simulink model "CubaModelTwoPoint"  (R2016a)
settings: Solver=FixedStepAuto  SolverMode=SingleTasking  StartTime=0.0  StopTime=5  FixedStep=0.001  RelTol=1e-3
values from neighbouring files (symbols this model uses):
  C_K = 2.1e-3    (= 0.0021)    [Init_TwoPoint.m]
  C_R = 2.1268e-5    (= 2.1268e-05)    [Init_TwoPoint.m]
  g = 9.81    [Init_TwoPoint.m]
  l_AB = 0.08455    [Init_TwoPoint.m]
  l_SA = 0.0751442    [Init_TwoPoint.m]
  m_K = 0.294    [Init_TwoPoint.m]
  m_R = 0.1298    [Init_TwoPoint.m]
  O_G_A = O_K_A + m_R * l_AB^2    (= 0.0042279015845)    [Init_TwoPoint.m]
  O_R_B = 0.088e-3    (= 8.8e-05)    [Init_TwoPoint.m]
  phi_K0 = degtorad(1)    [Init_TwoPoint.m]
  phi_K__d0 = degtorad(0)    [Init_TwoPoint.m]
  phi_R0 = degtorad(0)    [Init_TwoPoint.m]
  phi_R__d0 = degtorad(0)    [Init_TwoPoint.m]
  T_M_m = 12.4e-3    (= 0.0124)    [Init_TwoPoint.m]
undefined symbols (not defined in the file or in its folder): degtorad
libraries: simulink x1
settings Model: Creator=michael  LastModifiedBy=ich

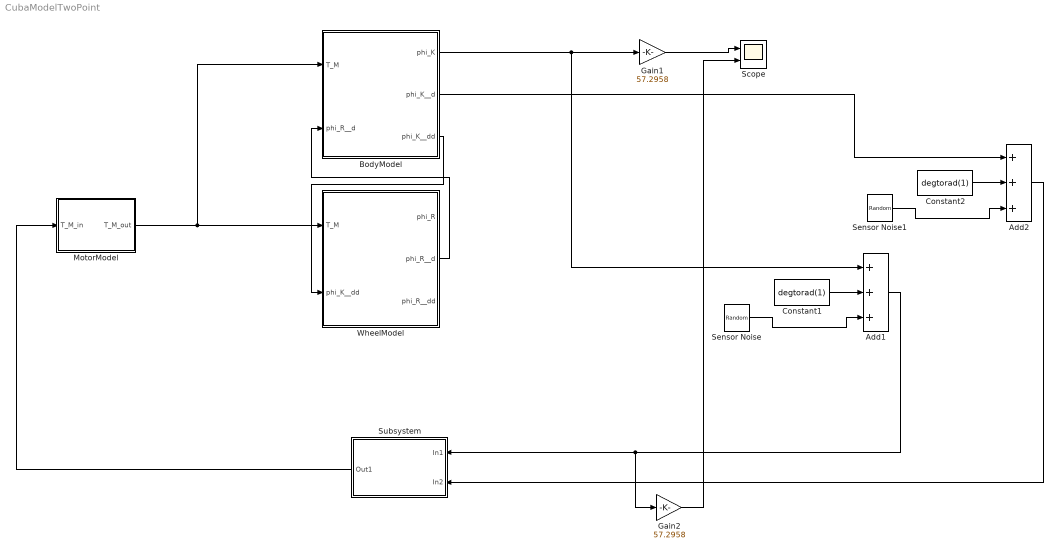
== system CubaModelTwoPoint ==
  Add1 : Sum  Inputs=+++
  Add2 : Sum  Inputs=+++
  BodyModel : Subsystem  SystemSampleTime=0.001
  Constant1 : Constant  Value=degtorad(1)  VectorParams1D=off
  Constant2 : Constant  Value=degtorad(1)  VectorParams1D=off
  Gain1 : Gain  Gain=57.2958
  Gain2 : Gain  Gain=57.2958
  "MotorModel " : Subsystem
  Scope : Scope  NumInputPorts=2
  Sensor Noise : UniformRandomNumber  Minimum=-0.0175  Maximum=0.0175  SampleTime=0.001
  Sensor Noise1 : UniformRandomNumber  Minimum=-0.0175  Maximum=0.0175  SampleTime=0.001
  Subsystem : Subsystem
  WheelModel : Subsystem  SystemSampleTime=0.001
  wires:
  BodyModel/3(phi_K__dd) -> WheelModel/2(phi_K__dd)
  "MotorModel "/1(T_M_out) -> BodyModel/1(T_M), WheelModel/1(T_M)
  BodyModel/1(phi_K) -> Add1/1, Gain1/1
  WheelModel/2(phi_R__d) -> BodyModel/2(phi_R__d)
  Gain1/1 -> Scope/1
  Gain2/1 -> Scope/2
  Add1/1 -> Gain2/1, Subsystem/1(In1)
  Constant1/1 -> Add1/2
  Sensor Noise/1 -> Add1/3
  Subsystem/1(Out1) -> "MotorModel "/1(T_M_in)
  Constant2/1 -> Add2/2
  Sensor Noise1/1 -> Add2/3
  BodyModel/2(phi_K__d) -> Add2/1
  Add2/1 -> Subsystem/2(In2)

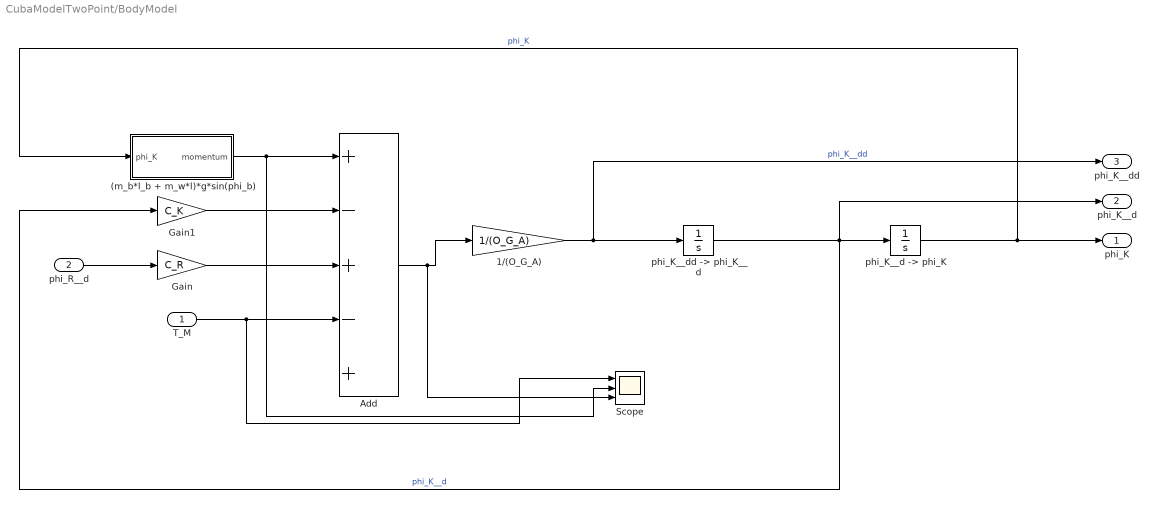
== system CubaModelTwoPoint/BodyModel ==
  T_M : Inport
  phi_R__d : Inport  Port=2
  (m_b*l_b + m_w*l)*g*sin(phi_b) : Subsystem
  1/(O_G_A) : Gain  Gain=1/(O_G_A)
  Add : Sum  Inputs=+-+-+
  Gain : Gain  Gain=C_R
  Gain1 : Gain  Gain=C_K
  Scope : Scope  NumInputPorts=3
  "phi_K__d -> phi_K" : Integrator  InitialCondition=phi_K0
  "phi_K__dd -> phi_K__d" : Integrator  InitialCondition=phi_K__d0
  phi_K : Outport
  phi_K__d : Outport  Port=2
  phi_K__dd : Outport  Port=3
  wires:
  T_M/1 -> Scope/1, Add/4
  Gain/1 -> Add/3
  Gain1/1 -> Add/2
  (m_b*l_b + m_w*l)*g*sin(phi_b)/1(momentum) -> Scope/2, Add/1
  phi_R__d/1 -> Gain/1
  Add/1 -> Scope/3, 1/(O_G_A)/1
  1/(O_G_A)/1 -> phi_K__dd/1, "phi_K__dd -> phi_K__d"/1  "phi_K__dd"
  "phi_K__dd -> phi_K__d"/1 -> Gain1/1, phi_K__d/1, "phi_K__d -> phi_K"/1  "phi_K__d"
  "phi_K__d -> phi_K"/1 -> phi_K/1, (m_b*l_b + m_w*l)*g*sin(phi_b)/1(phi_K)  "phi_K"

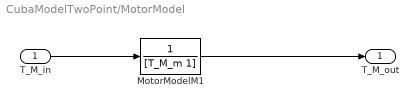
== system CubaModelTwoPoint/MotorModel  ==
  T_M_in : Inport
  MotorModelM1 : TransferFcn  Denominator=[T_M_m 1]
  T_M_out : Outport
  wires:
  T_M_in/1 -> MotorModelM1/1
  MotorModelM1/1 -> T_M_out/1

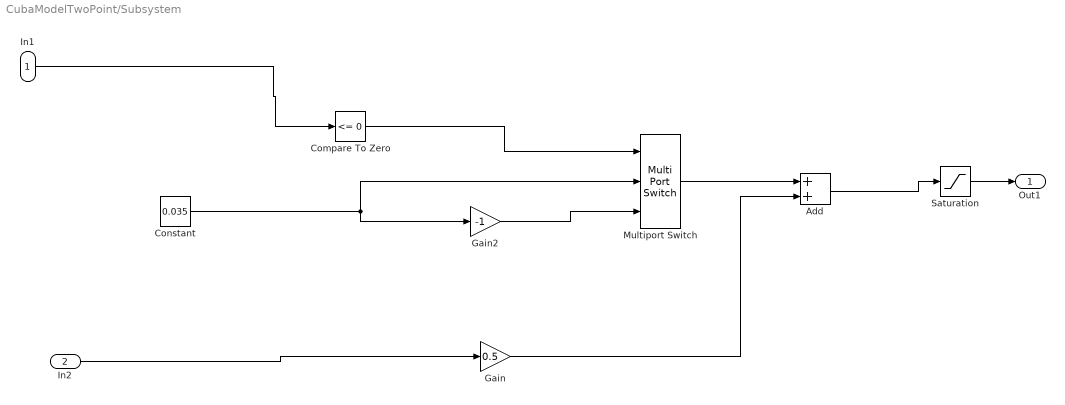
== system CubaModelTwoPoint/Subsystem ==
  In1 : Inport  SampleTime=0.02
  In2 : Inport  Port=2  SampleTime=0.02
  Add : Sum
  Compare To Zero : simulink/Logic and Bit Operations/Compare To Zero  relop=<=  OutDataTypeStr=boolean
  Constant : Constant  Value=0.035
  Gain : Gain  Gain=0.5
  Gain2 : Gain  Gain=-1
  Multiport Switch : MultiPortSwitch  DataPortOrder=Zero-based contiguous  Inputs=2
  Saturation : Saturate  UpperLimit=0.05  LowerLimit=-0.05
  Out1 : Outport
  wires:
  Constant/1 -> Gain2/1, Multiport Switch/2
  Gain2/1 -> Multiport Switch/3
  Compare To Zero/1 -> Multiport Switch/1
  Multiport Switch/1 -> Add/1
  Add/1 -> Saturation/1
  Gain/1 -> Add/2
  In2/1 -> Gain/1
  In1/1 -> Compare To Zero/1
  Saturation/1 -> Out1/1

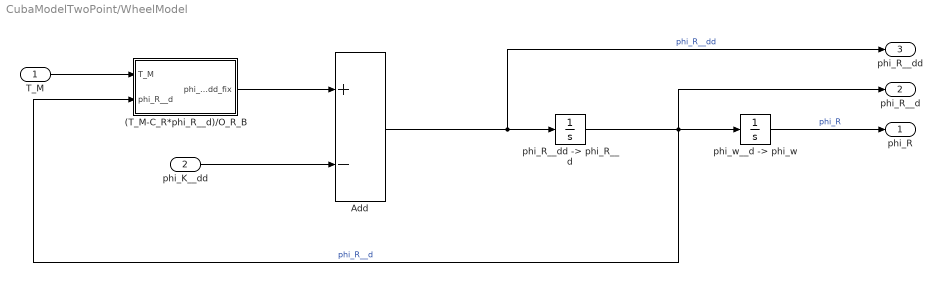
== system CubaModelTwoPoint/WheelModel ==
  T_M : Inport
  phi_K__dd : Inport  Port=2
  (T_M-C_R*phi_R__d)/O_R_B : Subsystem
  Add : Sum  Inputs=+-
  "phi_R__dd -> phi_R__d" : Integrator  InitialCondition=phi_R__d0
  "phi_w__d -> phi_w" : Integrator  InitialCondition=phi_R0
  phi_R : Outport
  phi_R__d : Outport  Port=2
  phi_R__dd : Outport  Port=3
  wires:
  phi_K__dd/1 -> Add/2
  Add/1 -> phi_R__dd/1, "phi_R__dd -> phi_R__d"/1  "phi_R__dd"
  "phi_R__dd -> phi_R__d"/1 -> phi_R__d/1, (T_M-C_R*phi_R__d)/O_R_B/2(phi_R__d), "phi_w__d -> phi_w"/1  "phi_R__d"
  (T_M-C_R*phi_R__d)/O_R_B/1(phi_R__dd_fix) -> Add/1
  T_M/1 -> (T_M-C_R*phi_R__d)/O_R_B/1(T_M)
  "phi_w__d -> phi_w"/1 -> phi_R/1  "phi_R"

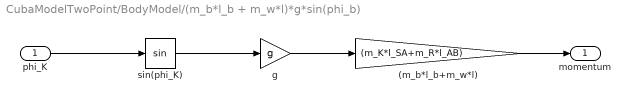
== system CubaModelTwoPoint/BodyModel/(m_b*l_b + m_w*l)*g*sin(phi_b) ==
  phi_K : Inport
  (m_b*l_b+m_w*l) : Gain  Gain=(m_K*l_SA+m_R*l_AB)
  g : Gain  Gain=g
  sin(phi_K) : Trigonometry
  momentum : Outport
  wires:
  sin(phi_K)/1 -> g/1
  phi_K/1 -> sin(phi_K)/1
  g/1 -> (m_b*l_b+m_w*l)/1
  (m_b*l_b+m_w*l)/1 -> momentum/1

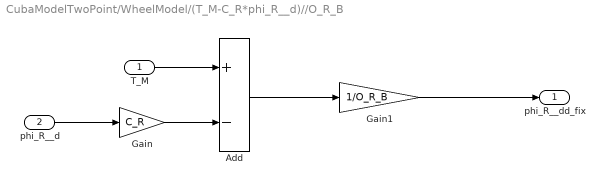
== system CubaModelTwoPoint/WheelModel/(T_M-C_R*phi_R__d)//O_R_B ==
  T_M : Inport
  phi_R__d : Inport  Port=2
  Add : Sum  Inputs=+-
  Gain : Gain  Gain=C_R
  Gain1 : Gain  Gain=1/O_R_B
  phi_R__dd_fix : Outport
  wires:
  T_M/1 -> Add/1
  phi_R__d/1 -> Gain/1
  Gain/1 -> Add/2
  Add/1 -> Gain1/1
  Gain1/1 -> phi_R__dd_fix/1
